simulink model "sim_esercitazione_3"  (R2025b)
settings: Solver=VariableStepAuto  StartTime=0.0  StopTime=t_sim  RelTol=1e-3
undefined symbols (not defined in the file): delta_d1, delta_d2, DiscIntNeverNeededParam, r, Ts
libraries: cstblocks x2
settings Model: Creator=giovannimasi  LastModifiedBy=giovannimasi

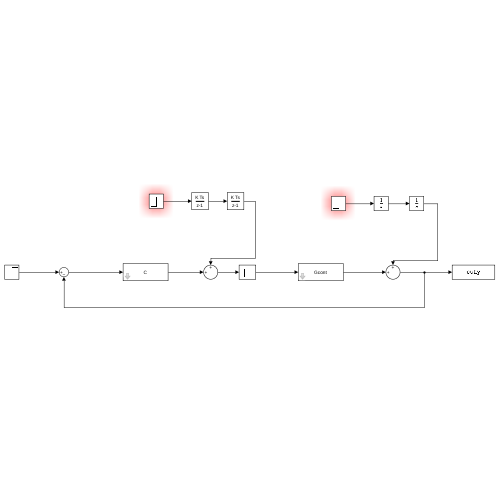
[thumbnail: Simulink's stored preview of the top-level diagram]
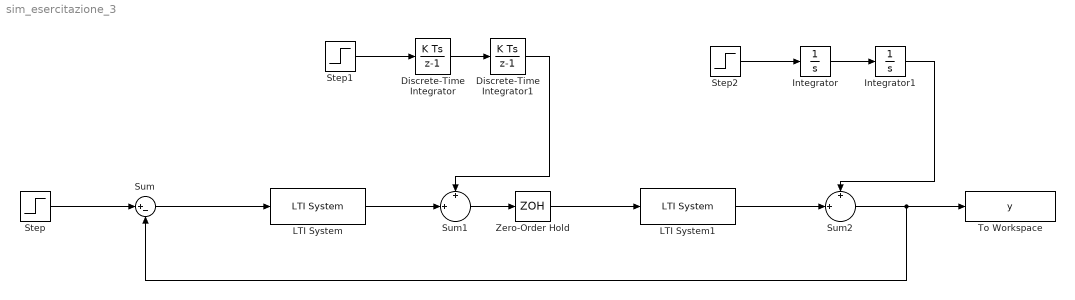
== system sim_esercitazione_3 ==
  Discrete-Time Integrator : DiscreteIntegrator  SampleTime=Ts  ICPrevOutput=DiscIntNeverNeededParam  ICPrevScaledInput=DiscIntNeverNeededParam
  Discrete-Time Integrator1 : DiscreteIntegrator  SampleTime=Ts  ICPrevOutput=DiscIntNeverNeededParam  ICPrevScaledInput=DiscIntNeverNeededParam
  Integrator : Integrator
  Integrator1 : Integrator
  LTI System : cstblocks/LTI System  sys=C  IC=[]  PadeOrder=0
  LTI System1 : cstblocks/LTI System  sys=Gcont  IC=[]  PadeOrder=0
  Step : Step  Time=0  After=r  SampleTime=Ts
  Step1 : Step  Time=0  After=delta_d1  SampleTime=Ts
  Step2 : Step  Time=0  After=delta_d2  SampleTime=Ts
  Sum : Sum  Inputs=|+-
  Sum1 : Sum  Inputs=+|+||
  Sum2 : Sum  Inputs=+|+||
  To Workspace : ToWorkspace  VariableName=y  SaveFormat=Timeseries  SampleTime=Ts
  Zero-Order Hold : ZeroOrderHold  SampleTime=-1
  wires:
  Step/1 -> Sum/1
  Sum/1 -> LTI System/1
  LTI System/1 -> Sum1/2
  Sum1/1 -> Zero-Order Hold/1
  LTI System1/1 -> Sum2/2
  Sum2/1 -> To Workspace/1, Sum/2
  Step1/1 -> Discrete-Time Integrator/1
  Discrete-Time Integrator/1 -> Discrete-Time Integrator1/1
  Discrete-Time Integrator1/1 -> Sum1/1
  Step2/1 -> Integrator/1
  Integrator/1 -> Integrator1/1
  Zero-Order Hold/1 -> LTI System1/1
  Integrator1/1 -> Sum2/1
